simulink model "LAB_1"  (R2024b)
settings: Solver=FixedStepAuto  StartTime=0.0  StopTime=10  FixedStep=0.01  RelTol=1e-3  EnableMultiTasking=on
libraries: stm32f4xxblockslib x1
settings Model: STM32="{\"AnalogInput\":[{\"ID\":\"untitled:2\"},{\"ID\":\"BasicKitP:2\"},{\"ID\":\"LAB_1:45\"}]}"  Creator=Chantouch  LastModifiedBy=chant
settings OptimizationCC: DefaultParameterBehavior=Inlined  EnhancedBackFolding=on  PassReuseOutputArgsAs=Individual arguments  ZeroExternalMemoryAtStartup=off  ZeroInternalMemoryAtStartup=off  MaxStackSize=512  OptimizeBlockOrder=speed  DifferentSizesBufferReuse=on  OptimizationCustomize=off  EfficientTunableParamExpr=on
settings DebuggingCC: ParameterTunabilityLossMsg=error
settings HardwareCC: ProdBitPerPointer=32  ProdBitPerSizeT=32  ProdBitPerPtrDiffT=32  ProdLargestAtomicInteger=Long  ProdLargestAtomicFloat=Double  ProdWordSize=32  ProdLongLongMode=on  ProdHWDeviceType=ARM Compatible->ARM Cortex-M
settings SFSimCC: MATLABDynamicMemAlloc=off
settings RTWCC: Description=Embedded Coder  SystemTargetFile=ert.tlc  HardwareBoard=STM32G4xx Based  TemplateMakefile=ert_default_tmf  Toolchain=GNU Tools for ARM Embedded Processors
settings CodeAppCC: ForceParamTrailComments=on  IgnoreCustomStorageClasses=off  OperatorAnnotations=on  SimulinkDataObjDesc=on  SFDataObjDesc=on  InsertBlockDesc=on
settings ERTTargetCC: TargetLangStandard=C99 (ISO)  CodeReplacementLibrary=ARM Cortex-M  ExtModeTransport=3  ExtModeStaticAlloc=on  ExtModeStaticAllocSize=2048  ExtModeMexFile=ext_xcp  ExtModeIntrfLevel=Level2 - Open

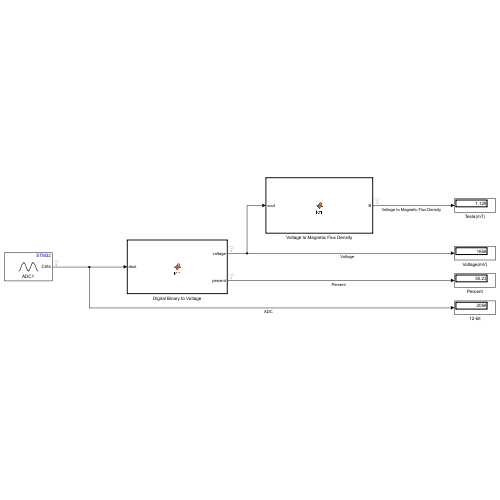
[thumbnail: Simulink's stored preview of the top-level diagram]
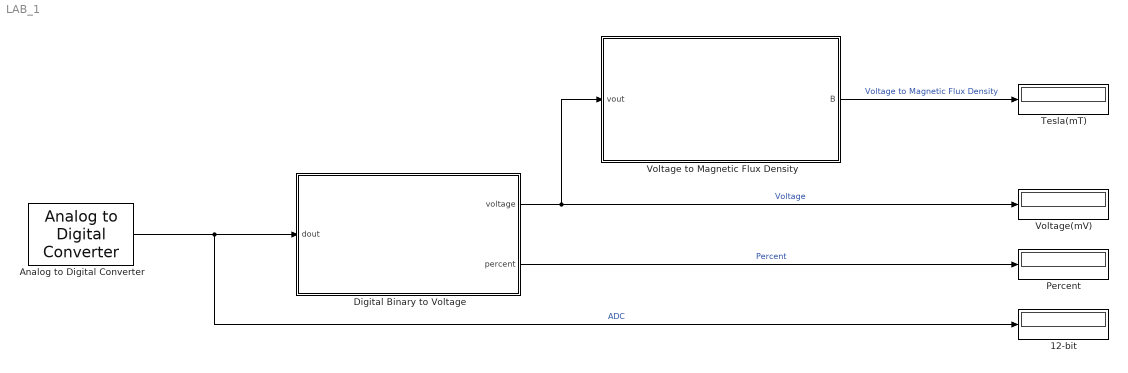
== system LAB_1 ==
  12-bit : Display
  Analog to Digital Converter : stm32f4xxblockslib/Analog to Digital Converter  ADCModule=ADC1  ConversionGroup=Regular  TriggerMode=Trigger and read  NumberOfConversions=1  EnableBufferConv=off  BufferLength=1  OutputStatus=off  SampleTime=-1  EnableSimPort=off  hoistedMaskSrc=ECSoC/ECSimCodegen/Analog to Digital Converter
  Digital Binary to Voltage : MATLAB Function  TreatAsAtomicUnit=on
  Percent : Display
      settings: Decimation=3
  Tesla(mT) : Display
  Voltage to Magnetic Flux Density : MATLAB Function  TreatAsAtomicUnit=on
  Voltage(mV) : Display
      settings: Decimation=3
  wires:
  Analog to Digital Converter/1 -> 12-bit/1, Digital Binary to Voltage/1(dout)  "ADC"
  Digital Binary to Voltage/1(voltage) -> Voltage to Magnetic Flux Density/1(vout), Voltage(mV)/1  "Voltage"
  Digital Binary to Voltage/2(percent) -> Percent/1  "Percent"
  Voltage to Magnetic Flux Density/1(B) -> Tesla(mT)/1  "Voltage to Magnetic Flux Density"

== matlab function LAB_1/Voltage to Magnetic Flux Density ==
  data: vout input; B output
function B = Calculations(vout)

    % คำนวณหา Magnetic flux density (B)
    % Output Voltage = V_Q + B * (Sensitivity * (1 + S_TC * (T_A - 25)))
    raw_B = (double(vout/1000) - 1.650) / (7.5 * (1 + 0.0012 * (25 - 25)));
    B = raw_B * 1000;
    
end

== matlab function LAB_1/Digital Binary to Voltage ==
  data: dout input; voltage output; percent output
function [voltage, percent] = Calculations(dout)

    vin = double(dout)/(2^12 - 1)*3.3; % Input Voltage คือ (Digital Output / จำนวนบิต - 1) * Reference Voltage
    voltage = double(vin)*1000; % แปลง Volts เป็น milliVolts
    percent = (double(vin)/3.3)*100; % Percent คือ (Input Voltage / 3.3) * 100

end
